simulink model "exo1"  (R2020b)
settings: Solver=VariableStepAuto  StartTime=0.0  StopTime=10.0  RelTol=1e-3
values from neighbouring files (symbols this model uses):
  Te = 1/fe    [bandwidth_calc.m]    (also in exo1_mfile.m)
settings Model: Creator=alex  LastModifiedBy=alex

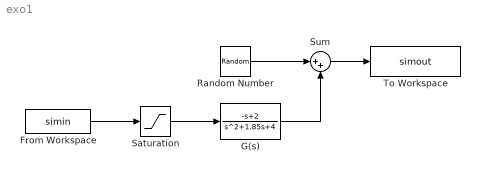
== system exo1 ==
  From Workspace : FromWorkspace  VariableName=simin  SampleTime=Te
  G(s) : TransferFcn  Numerator=[-1 2]  Denominator=[1 1.85 4]
  Random Number : RandomNumber  Variance=0.01  SampleTime=Te
  Saturation : Saturate
  Sum : Sum  Inputs=|++
  To Workspace : ToWorkspace  VariableName=simout  SaveFormat=Timeseries  SampleTime=Te
  wires:
  Saturation/1 -> G(s)/1
  Random Number/1 -> Sum/1
  G(s)/1 -> Sum/2
  From Workspace/1 -> Saturation/1
  Sum/1 -> To Workspace/1
